simulink model "gm_sampleModel1785_3_sub"  (R2023a)
settings: Solver=VariableStepAuto  StartTime=0.0  StopTime=10.0  RelTol=1e-3
libraries: simulink x2, hdlsllib x1
settings Model: Creator=user1  LastModifiedBy=user1
settings OptimizationCC: BlockReduction=off  ConditionallyExecuteInputs=off
settings DebuggingCC: InheritedTsInSrcMsg=none

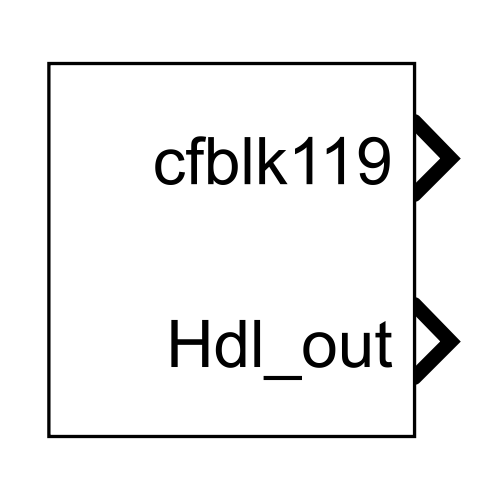
[thumbnail: Simulink's stored preview of the top-level diagram]
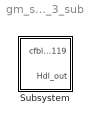
== system gm_sampleModel1785_3_sub ==
  Subsystem : Subsystem

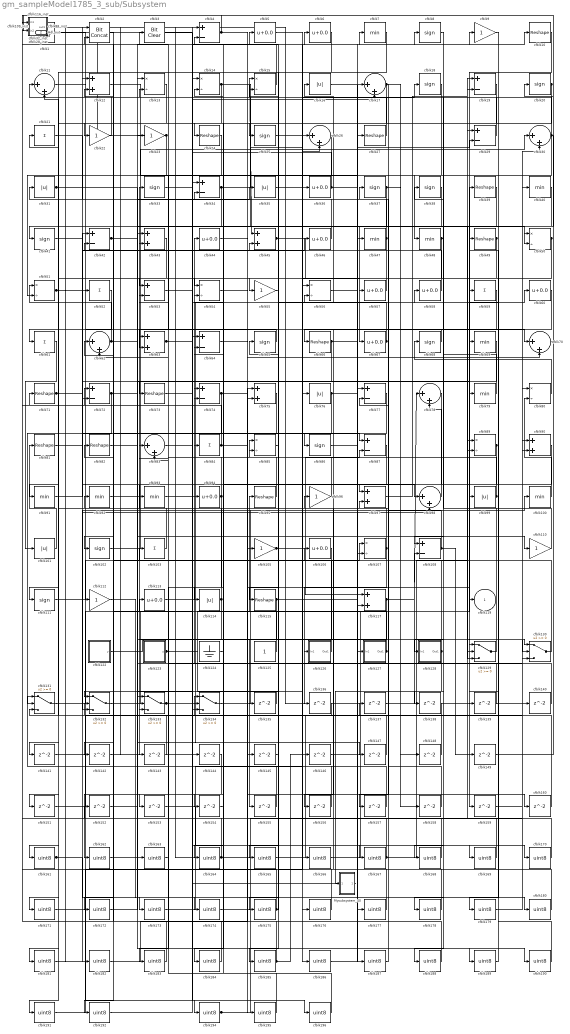
== system gm_sampleModel1785_3_sub/Subsystem ==
  Mysubsystem_40 : Subsystem
  cfblk1 : simulink/Logic and Bit Operations/Bit Clear  iBit=0
      settings: LibrarySourceBlock=|
      | hdlsllib/Logic and Bit
      | Operations/Bit Clear
  cfblk{10,24,27,39,49,66,71,73,81..82,95,115} (12 alike) : Reshape
  cfblk{7,40,47..48,69,79,91..93,100} (10 alike) : MinMax  OutDataTypeStr=uint8
  cfblk{16,31,35,76,99,101,114} (7 alike) : Abs  OutDataTypeStr=uint8  SaturateOnIntegerOverflow=off
  cfblk{8,18,20,25,33,37..38,41,65,68,86,102,111} (13 alike) : Signum
  cfblk{21,52,59,61,84,103} (6 alike) : Sum  Inputs=+  OutDataTypeStr=uint8
  cfblk{9,22..23,55,96,105,110,112} (8 alike) : Gain  OutDataTypeStr=uint8
  cfblk{5..6,36,44,46,57..58,60,67,94,106,113} (12 alike) : Bias  Bias=0.0  SaturateOnIntegerOverflow=off
  cfblk{13..15,50..51,54,56,80,85,89,107} (11 alike) : Product  Inputs=*/  OutDataTypeStr=uint8  RndMeth=Zero  SaturateOnIntegerOverflow=on
  cfblk{4,19,29,34,42,53,64,72,74,77,87,108} (12 alike) : Sum  Inputs=+-  OutDataTypeStr=uint8
  cfblk109_inst : Subsystem
  cfblk{11,17,26,30,62,70,78,83,98} (9 alike) : Sum  Inputs=|++  OutDataTypeStr=uint8
  cfblk116_inst : Subsystem
  cfblk{12,43,45,63,75,90,97,117} (8 alike) : Sum  OutDataTypeStr=uint8
  cfblk122 : Subsystem  mask(Counter Limited){uplimit=double(7), tsamp=double(-1)}
      mask prompts: uplimit "Simulink:masks:UpperLimit_MP"; tsamp "Simulink:masks:SampleTime_MP"
      mask help: Simulink:masks:CounterLimited_MD
      mask init:
      | nbits = double(8);
      | tsamp = double(-1);
      | uplimit = double(7);
  cfblk123 : Subsystem  mask(Counter Free-Running){NumBits=double(16), tsamp=double(-1)}
      mask prompts: NumBits "Simulink:masks:NumberOfBits_MP"; tsamp "Simulink:masks:SampleTime_MP"
      mask help: Simulink:masks:CounterFreeRunning_MD
  cfblk124 : Ground
  cfblk125 : Constant  OutDataTypeStr=uint8  SampleTime=-1
  cfblk126 : Subsystem
  cfblk127 : Subsystem
  cfblk128 : Subsystem
  cfblk{129..134} (6 alike) : Switch  OutDataTypeStr=uint8  SaturateOnIntegerOverflow=off  InputSameDT=off
  cfblk{135..149,151..160} (25 alike) : Delay  SampleTime=1
  cfblk{161..192,194..196} (35 alike) : DataTypeConversion  OutDataTypeStr=uint8  SaturateOnIntegerOverflow=off  RndMeth=Floor
  cfblk2 : hdlsllib/Logic and Bit Operations/Bit Concat  numInputs=2
  cfblk28_inst : Subsystem
  cfblk3 : simulink/Logic and Bit Operations/Bit Clear  iBit=0
      settings: LibrarySourceBlock=|
      | hdlsllib/Logic and Bit
      | Operations/Bit Clear
  cfblk32_inst : Subsystem
  cfblk88_inst : Subsystem
  cfblk119 : Outport  OutDataTypeStr=uint8  SampleTime=1  VectorParamsAs1DForOutWhenUnconnected=off
  Hdl_out : Outport  Port=2  OutDataTypeStr=uint8  SampleTime=1
  wires:
  Mysubsystem_40/1(Out1) -> cfblk1/1
  cfblk1/1 -> cfblk194/1
  cfblk10/1 -> cfblk159/1
  cfblk100/1 -> cfblk80/2
  cfblk101/1 -> cfblk81/1
  cfblk102/1 -> cfblk30/1
  cfblk103/1 -> cfblk33/1
  cfblk105/1 -> cfblk87/2, cfblk117/1
  cfblk106/1 -> cfblk136/1
  cfblk107/1 -> cfblk126/1(In1), cfblk92/1
  cfblk108/1 -> cfblk37/1, cfblk149/1
  cfblk109_inst/1(out1) -> cfblk140/1
  cfblk11/1 -> cfblk143/1
  cfblk110/1 -> cfblk15/1
  cfblk111/1 -> cfblk107/1
  cfblk112/1 -> cfblk180/1
  cfblk113/1 -> cfblk44/1
  cfblk114/1 -> cfblk31/1, cfblk153/1
  cfblk115/1 -> cfblk60/1, cfblk155/1
  cfblk116_inst/1(out1) -> cfblk144/1
  cfblk117/1 -> cfblk78/1, cfblk133/3
  cfblk12/1 -> cfblk177/1
  cfblk122/1(y) -> cfblk130/1
  cfblk123/1(y) -> cfblk39/1, cfblk176/1
  cfblk124/1 -> cfblk4/2
  cfblk125/1 -> cfblk82/1
  cfblk126/1(Out1) -> cfblk62/1
  cfblk127/1(Out1) -> cfblk95/1, cfblk42/2
  cfblk128/1(Out1) -> Mysubsystem_40/1(In1), cfblk103/1
  cfblk129/1 -> cfblk69/1
  cfblk13/1 -> cfblk181/1
  cfblk130/1 -> cfblk106/1
  cfblk131/1 -> cfblk113/1
  cfblk132/1 -> cfblk34/1
  cfblk133/1 -> cfblk58/1, cfblk187/1
  cfblk134/1 -> cfblk100/1
  cfblk135/1 -> cfblk132/1
  cfblk136/1 -> cfblk132/2
  cfblk137/1 -> cfblk108/2
  cfblk138/1 -> cfblk131/3
  cfblk139/1 -> cfblk53/2
  cfblk14/1 -> cfblk45/1, cfblk129/3, cfblk61/1
  cfblk140/1 -> cfblk74/1
  cfblk141/1 -> cfblk89/2
  cfblk142/1 -> cfblk129/2
  cfblk143/1 -> cfblk51/1
  cfblk144/1 -> cfblk162/1
  cfblk145/1 -> cfblk45/2
  cfblk146/1 -> cfblk19/2
  cfblk147/1 -> cfblk64/2
  cfblk148/1 -> cfblk12/2
  cfblk149/1 -> cfblk88_inst/2(in2)
  cfblk15/1 -> cfblk4/1
  cfblk151/1 -> cfblk30/2
  cfblk152/1 -> cfblk34/2
  cfblk153/1 -> cfblk169/1
  cfblk154/1 -> cfblk134/1
  cfblk155/1 -> cfblk72/1
  cfblk156/1 -> cfblk131/1
  cfblk157/1 -> cfblk14/2
  cfblk158/1 -> cfblk97/2
  cfblk159/1 -> cfblk80/1
  cfblk16/1 -> cfblk127/1(In1)
  cfblk160/1 -> cfblk54/2
  cfblk161/1 -> cfblk99/1, cfblk173/1
  cfblk162/1 -> cfblk43/1
  cfblk163/1 -> cfblk43/2
  cfblk164/1 -> cfblk75/2, cfblk2/2, cfblk116_inst/2(in2)
  cfblk165/1 -> cfblk90/1
  cfblk166/1 -> cfblk90/2
  cfblk167/1 -> cfblk32_inst/1(in1), cfblk29/1
  cfblk168/1 -> cfblk83/1
  cfblk169/1 -> cfblk83/2
  cfblk17/1 -> cfblk184/1, cfblk158/1, cfblk157/1
  cfblk170/1 -> cfblk89/1
  cfblk171/1 -> cfblk93/1
  cfblk172/1 -> cfblk6/1
  cfblk173/1 -> cfblk26/1
  cfblk174/1 -> cfblk26/2
  cfblk175/1 -> cfblk88_inst/1(in1), cfblk65/1
  cfblk176/1 -> cfblk85/1
  cfblk177/1 -> cfblk85/2
  cfblk178/1 -> cfblk137/1
  cfblk179/1 -> cfblk40/1
  cfblk18/1 -> cfblk48/1
  cfblk180/1 -> cfblk96/1
  cfblk181/1 -> cfblk112/1
  cfblk182/1 -> cfblk105/1
  cfblk183/1 -> cfblk28_inst/1(in1)
  cfblk184/1 -> cfblk28_inst/2(in2)
  cfblk185/1 -> cfblk109_inst/2(in2), cfblk146/1
  cfblk186/1 -> cfblk77/1
  cfblk187/1 -> cfblk77/2
  cfblk188/1 -> cfblk152/1
  cfblk189/1 -> cfblk59/1
  cfblk19/1 -> cfblk102/1
  cfblk190/1 -> cfblk49/1
  cfblk191/1 -> cfblk56/1
  cfblk192/1 -> cfblk56/2
  cfblk194/1 -> cfblk36/1, cfblk17/1, cfblk130/3
  cfblk195/1 -> cfblk3/1
  cfblk196/1 -> cfblk84/1
  cfblk2/1 -> cfblk22/1
  cfblk20/1 -> cfblk25/1, cfblk139/1, cfblk138/1
  cfblk21/1 -> cfblk98/1
  cfblk22/1 -> cfblk11/1
  cfblk23/1 -> cfblk51/2, Hdl_out/1
  cfblk24/1 -> cfblk63/2
  cfblk25/1 -> cfblk9/1
  cfblk26/1 -> cfblk172/1
  cfblk27/1 -> cfblk5/1
  cfblk28_inst/1(out1) -> cfblk182/1
  cfblk29/1 -> cfblk12/1
  cfblk3/1 -> cfblk196/1
  cfblk30/1 -> cfblk24/1, cfblk114/1, cfblk50/2, cfblk13/2
  cfblk31/1 -> cfblk189/1, cfblk50/1
  cfblk32_inst/1(out1) -> cfblk166/1
  cfblk33/1 -> cfblk70/1
  cfblk34/1 -> cfblk72/2, cfblk7/1
  cfblk35/1 -> cfblk18/1
  cfblk36/1 -> cfblk29/2, cfblk14/1
  cfblk37/1 -> cfblk67/1, cfblk148/1
  cfblk38/1 -> cfblk111/1
  cfblk39/1 -> cfblk41/1
  cfblk4/1 -> cfblk70/2, cfblk109_inst/1(in1)
  cfblk40/1 -> cfblk178/1
  cfblk41/1 -> cfblk86/1
  cfblk42/1 -> cfblk23/1, cfblk147/1
  cfblk43/1 -> cfblk161/1
  cfblk44/1 -> cfblk97/1
  cfblk45/1 -> cfblk76/1, cfblk117/2
  cfblk46/1 -> cfblk21/1
  cfblk47/1 -> cfblk2/1, cfblk91/1
  cfblk48/1 -> cfblk171/1, cfblk128/1(In1)
  cfblk49/1 -> cfblk132/3, cfblk55/1
  cfblk5/1 -> cfblk57/1
  cfblk50/1 -> cfblk53/1, cfblk151/1
  cfblk51/1 -> cfblk186/1, cfblk163/1, cfblk145/1
  cfblk52/1 -> cfblk191/1
  cfblk53/1 -> cfblk64/1
  cfblk54/1 -> cfblk195/1
  cfblk55/1 -> cfblk165/1
  cfblk56/1 -> cfblk190/1
  cfblk57/1 -> cfblk54/1
  cfblk58/1 -> cfblk13/1
  cfblk59/1 -> cfblk188/1
  cfblk6/1 -> cfblk141/1
  cfblk60/1 -> cfblk156/1
  cfblk61/1 -> cfblk101/1
  cfblk62/1 -> cfblk133/1, cfblk11/2, cfblk110/1
  cfblk63/1 -> cfblk94/1, cfblk17/2
  cfblk64/1 -> cfblk129/1
  cfblk65/1 -> cfblk63/1
  cfblk66/1 -> cfblk8/1, cfblk133/2, cfblk10/1
  cfblk67/1 -> cfblk16/1, cfblk15/2
  cfblk68/1 -> cfblk66/1
  cfblk69/1 -> cfblk73/1
  cfblk7/1 -> cfblk135/1
  cfblk70/1 -> cfblk20/1
  cfblk71/1 -> cfblk87/1, cfblk79/1
  cfblk72/1 -> cfblk131/2, cfblk130/2
  cfblk73/1 -> cfblk35/1
  cfblk74/1 -> cfblk134/2, cfblk119/1
  cfblk75/1 -> cfblk142/1
  cfblk76/1 -> cfblk27/1, cfblk192/1
  cfblk77/1 -> cfblk185/1
  cfblk78/1 -> cfblk115/1
  cfblk79/1 -> cfblk38/1
  cfblk8/1 -> cfblk168/1
  cfblk80/1 -> cfblk68/1
  cfblk81/1 -> cfblk98/2
  cfblk82/1 -> cfblk134/3
  cfblk83/1 -> cfblk167/1
  cfblk84/1 -> cfblk74/2, cfblk116_inst/1(in1), cfblk160/1
  cfblk85/1 -> cfblk175/1
  cfblk86/1 -> cfblk47/1
  cfblk87/1 -> cfblk154/1
  cfblk88_inst/1(out1) -> cfblk52/1
  cfblk89/1 -> cfblk108/1, cfblk107/2
  cfblk9/1 -> cfblk179/1
  cfblk90/1 -> cfblk164/1
  cfblk91/1 -> cfblk46/1
  cfblk92/1 -> cfblk174/1
  cfblk93/1 -> cfblk170/1
  cfblk94/1 -> cfblk71/1, cfblk183/1
  cfblk95/1 -> cfblk62/2
  cfblk96/1 -> cfblk42/1
  cfblk97/1 -> cfblk19/1
  cfblk98/1 -> cfblk78/2
  cfblk99/1 -> cfblk75/1, cfblk32_inst/2(in2)

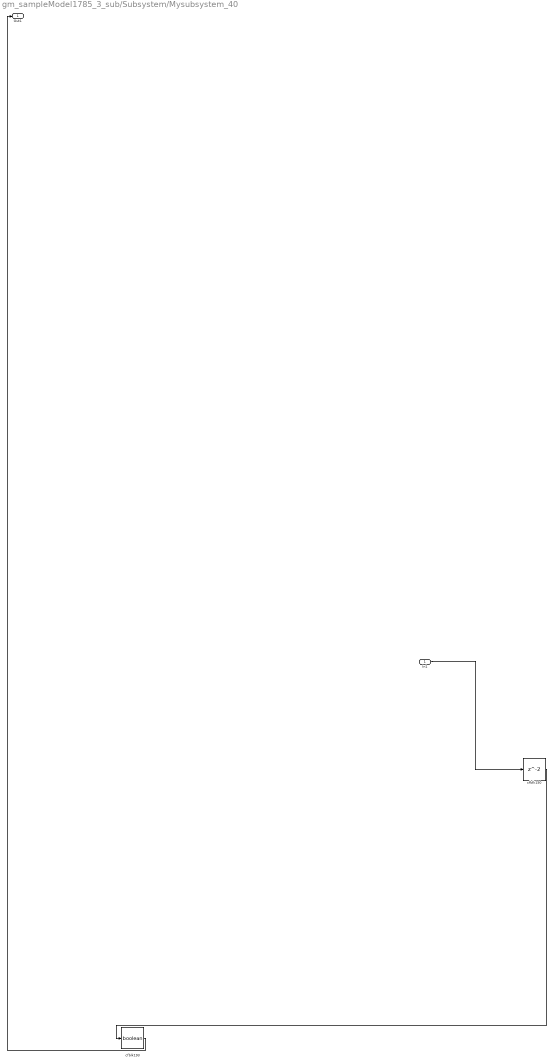
== system gm_sampleModel1785_3_sub/Subsystem/Mysubsystem_40 ==
  In1 : Inport  OutDataTypeStr=uint8  PortDimensions=1  SampleTime=1
  cfblk150 : Delay  SampleTime=1
  cfblk193 : DataTypeConversion  OutDataTypeStr=boolean  SaturateOnIntegerOverflow=off  RndMeth=Floor
  Out1 : Outport  SampleTime=1
  wires:
  In1/1 -> cfblk150/1
  cfblk150/1 -> cfblk193/1
  cfblk193/1 -> Out1/1

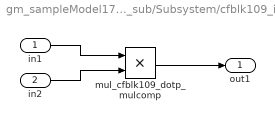
== system gm_sampleModel1785_3_sub/Subsystem/cfblk109_inst ==
  in1 : Inport  OutDataTypeStr=uint8  SampleTime=1
  in2 : Inport  Port=2  OutDataTypeStr=uint8  SampleTime=1
  mul_cfblk109_dotp_mulcomp : Product  Inputs=**  OutDataTypeStr=uint8  SampleTime=1
  out1 : Outport  OutDataTypeStr=uint8  SampleTime=1
  wires:
  in1/1 -> mul_cfblk109_dotp_mulcomp/1
  in2/1 -> mul_cfblk109_dotp_mulcomp/2
  mul_cfblk109_dotp_mulcomp/1 -> out1/1

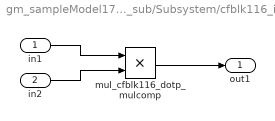
== system gm_sampleModel1785_3_sub/Subsystem/cfblk116_inst ==
  in1 : Inport  OutDataTypeStr=uint8  SampleTime=1
  in2 : Inport  Port=2  OutDataTypeStr=uint8  SampleTime=1
  mul_cfblk116_dotp_mulcomp : Product  Inputs=**  OutDataTypeStr=uint8  SampleTime=1
  out1 : Outport  OutDataTypeStr=uint8  SampleTime=1
  wires:
  in1/1 -> mul_cfblk116_dotp_mulcomp/1
  in2/1 -> mul_cfblk116_dotp_mulcomp/2
  mul_cfblk116_dotp_mulcomp/1 -> out1/1

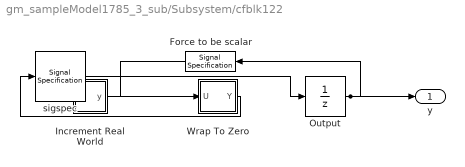
== system gm_sampleModel1785_3_sub/Subsystem/cfblk122 ==
  Force to be scalar : SignalSpecification  DisableCoverage=on  Dimensions=1
  Increment Real World : Subsystem  mask(Real World Value Increment){}
      mask help: Simulink:masks:RealWorldValueIncrement_MD
      mask Display: disp('V++')
  Output : UnitDelay  InitialCondition=0.0  SampleTime=tsamp  HasFrameUpgradeWarning=on
  Wrap To Zero : Subsystem  mask(Wrap To Zero){Threshold=double(7)}
      mask prompts: Threshold "Simulink:masks:Threshold_MP"
      mask help: Simulink:masks:WrapToZero_MD
  sigspec : SignalSpecification  OutDataTypeStr=uint8  Dimensions=1
  y : Outport  SampleTime=1
  wires:
  Force to be scalar/1 -> Increment Real World/1(u)
  Increment Real World/1(y) -> Wrap To Zero/1(U)
  Output/1 -> Force to be scalar/1, y/1
  Wrap To Zero/1(Y) -> sigspec/1
  sigspec/1 -> Output/1

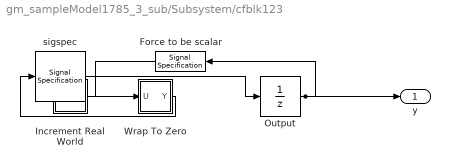
== system gm_sampleModel1785_3_sub/Subsystem/cfblk123 ==
  Force to be scalar : SignalSpecification  DisableCoverage=on  Dimensions=1
  Increment Real World : Subsystem  mask(Real World Value Increment){}
      mask help: Simulink:masks:RealWorldValueIncrement_MD
      mask Display: disp('V++')
  Output : UnitDelay  InitialCondition=0.0  SampleTime=tsamp  HasFrameUpgradeWarning=on
  Wrap To Zero : Subsystem  mask(Wrap To Zero){Threshold=double(65535)}
      mask prompts: Threshold "Simulink:masks:Threshold_MP"
      mask help: Simulink:masks:WrapToZero_MD
  sigspec : SignalSpecification  OutDataTypeStr=uint16  Dimensions=1
  y : Outport  SampleTime=1
  wires:
  Force to be scalar/1 -> Increment Real World/1(u)
  Increment Real World/1(y) -> Wrap To Zero/1(U)
  Output/1 -> Force to be scalar/1, y/1
  Wrap To Zero/1(Y) -> sigspec/1
  sigspec/1 -> Output/1

== system gm_sampleModel1785_3_sub/Subsystem/cfblk126 ==
  In1 : Inport  OutDataTypeStr=uint8  PortDimensions=1  SampleTime=1
  Out1 : Outport  SampleTime=1
  wires:
  In1/1 -> Out1/1

== system gm_sampleModel1785_3_sub/Subsystem/cfblk127 ==
  In1 : Inport  OutDataTypeStr=uint8  PortDimensions=1  SampleTime=1
  Out1 : Outport  SampleTime=1
  wires:
  In1/1 -> Out1/1

== system gm_sampleModel1785_3_sub/Subsystem/cfblk128 ==
  In1 : Inport  OutDataTypeStr=uint8  PortDimensions=1  SampleTime=1
  Out1 : Outport  SampleTime=1
  wires:
  In1/1 -> Out1/1

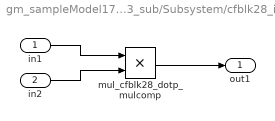
== system gm_sampleModel1785_3_sub/Subsystem/cfblk28_inst ==
  in1 : Inport  OutDataTypeStr=uint8  SampleTime=1
  in2 : Inport  Port=2  OutDataTypeStr=uint8  SampleTime=1
  mul_cfblk28_dotp_mulcomp : Product  Inputs=**  OutDataTypeStr=uint8  SampleTime=1
  out1 : Outport  OutDataTypeStr=uint8  SampleTime=1
  wires:
  in1/1 -> mul_cfblk28_dotp_mulcomp/1
  in2/1 -> mul_cfblk28_dotp_mulcomp/2
  mul_cfblk28_dotp_mulcomp/1 -> out1/1

== system gm_sampleModel1785_3_sub/Subsystem/cfblk32_inst ==
  in1 : Inport  OutDataTypeStr=uint8  SampleTime=1
  in2 : Inport  Port=2  OutDataTypeStr=uint8  SampleTime=1
  mul_cfblk32_dotp_mulcomp : Product  Inputs=**  OutDataTypeStr=uint8  SampleTime=1
  out1 : Outport  OutDataTypeStr=uint8  SampleTime=1
  wires:
  in1/1 -> mul_cfblk32_dotp_mulcomp/1
  in2/1 -> mul_cfblk32_dotp_mulcomp/2
  mul_cfblk32_dotp_mulcomp/1 -> out1/1

== system gm_sampleModel1785_3_sub/Subsystem/cfblk88_inst ==
  in1 : Inport  OutDataTypeStr=uint8  SampleTime=1
  in2 : Inport  Port=2  OutDataTypeStr=uint8  SampleTime=1
  mul_cfblk88_dotp_mulcomp : Product  Inputs=**  OutDataTypeStr=uint8  SampleTime=1
  out1 : Outport  OutDataTypeStr=uint8  SampleTime=1
  wires:
  in1/1 -> mul_cfblk88_dotp_mulcomp/1
  in2/1 -> mul_cfblk88_dotp_mulcomp/2
  mul_cfblk88_dotp_mulcomp/1 -> out1/1

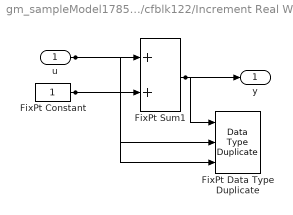
== system gm_sampleModel1785_3_sub/Subsystem/cfblk122/Increment Real World ==
  u : Inport  OutDataTypeStr=uint8  SampleTime=1
  FixPt Constant : Constant  DisableCoverage=on  OutDataTypeStr=Inherit: Inherit via back propagation  SampleTime=-1
  FixPt Data Type Duplicate : DataTypeDuplicate  DisableCoverage=on  NumInputPorts=3
  FixPt Sum1 : Sum  InputSameDT=on  OutDataTypeStr=Inherit: Inherit via back propagation  LockScale=on
  y : Outport  SampleTime=1
  wires:
  u/1 -> FixPt Sum1/1, FixPt Data Type Duplicate/2
  FixPt Constant/1 -> FixPt Sum1/2, FixPt Data Type Duplicate/3
  FixPt Sum1/1 -> FixPt Data Type Duplicate/1, y/1

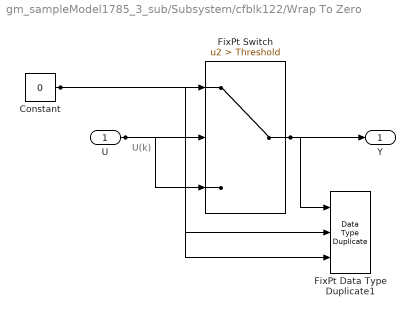
== system gm_sampleModel1785_3_sub/Subsystem/cfblk122/Wrap To Zero ==
  note: U(k)
  U : Inport  OutDataTypeStr=uint8  SampleTime=1
  Constant : Constant  DisableCoverage=on  Value=0  OutDataTypeStr=Inherit: Inherit via back propagation  SampleTime=-1
  FixPt Data Type Duplicate1 : DataTypeDuplicate  DisableCoverage=on  NumInputPorts=3
  FixPt Switch : Switch  Criteria=u2 > Threshold  Threshold=Threshold  OutDataTypeStr=Inherit: Inherit via back propagation  ZeroCross=off  SaturateOnIntegerOverflow=off  InputSameDT=off
  Y : Outport  SampleTime=1
  wires:
  U/1 -> FixPt Switch/3, FixPt Switch/2, FixPt Data Type Duplicate1/2
  Constant/1 -> FixPt Switch/1, FixPt Data Type Duplicate1/3
  FixPt Switch/1 -> FixPt Data Type Duplicate1/1, Y/1

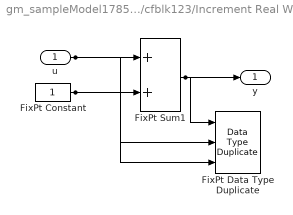
== system gm_sampleModel1785_3_sub/Subsystem/cfblk123/Increment Real World ==
  u : Inport  OutDataTypeStr=uint16  SampleTime=1
  FixPt Constant : Constant  DisableCoverage=on  OutDataTypeStr=Inherit: Inherit via back propagation  SampleTime=-1
  FixPt Data Type Duplicate : DataTypeDuplicate  DisableCoverage=on  NumInputPorts=3
  FixPt Sum1 : Sum  InputSameDT=on  OutDataTypeStr=Inherit: Inherit via back propagation  LockScale=on
  y : Outport  SampleTime=1
  wires:
  u/1 -> FixPt Sum1/1, FixPt Data Type Duplicate/2
  FixPt Constant/1 -> FixPt Sum1/2, FixPt Data Type Duplicate/3
  FixPt Sum1/1 -> FixPt Data Type Duplicate/1, y/1

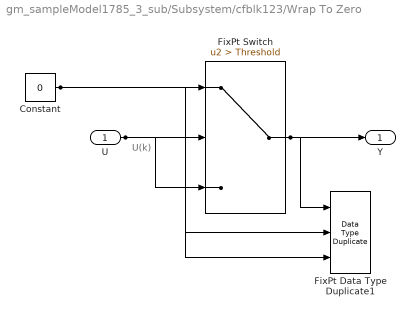
== system gm_sampleModel1785_3_sub/Subsystem/cfblk123/Wrap To Zero ==
  note: U(k)
  U : Inport  OutDataTypeStr=uint16  SampleTime=1
  Constant : Constant  DisableCoverage=on  Value=0  OutDataTypeStr=Inherit: Inherit via back propagation  SampleTime=-1
  FixPt Data Type Duplicate1 : DataTypeDuplicate  DisableCoverage=on  NumInputPorts=3
  FixPt Switch : Switch  Criteria=u2 > Threshold  Threshold=Threshold  OutDataTypeStr=Inherit: Inherit via back propagation  ZeroCross=off  SaturateOnIntegerOverflow=off  InputSameDT=off
  Y : Outport  SampleTime=1
  wires:
  U/1 -> FixPt Switch/3, FixPt Switch/2, FixPt Data Type Duplicate1/2
  Constant/1 -> FixPt Switch/1, FixPt Data Type Duplicate1/3
  FixPt Switch/1 -> FixPt Data Type Duplicate1/1, Y/1
